simulink model "simulink6"  (R2025b)
settings: Solver=ode45  StartTime=0.0  StopTime=50  MaxStep=2^-5  RelTol=1e-3
settings Model: Creator=mizula  LastModifiedBy=mizula

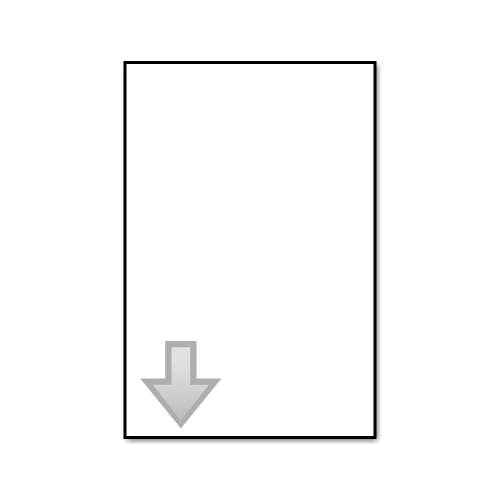
[thumbnail: Simulink's stored preview of the top-level diagram]
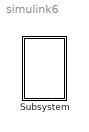
== system simulink6 ==
  Subsystem : Subsystem  mask{g=9.81, m1=1, m2=3, M=1, R=0.001, r0=2, th0=90, r1=0, th1=0}

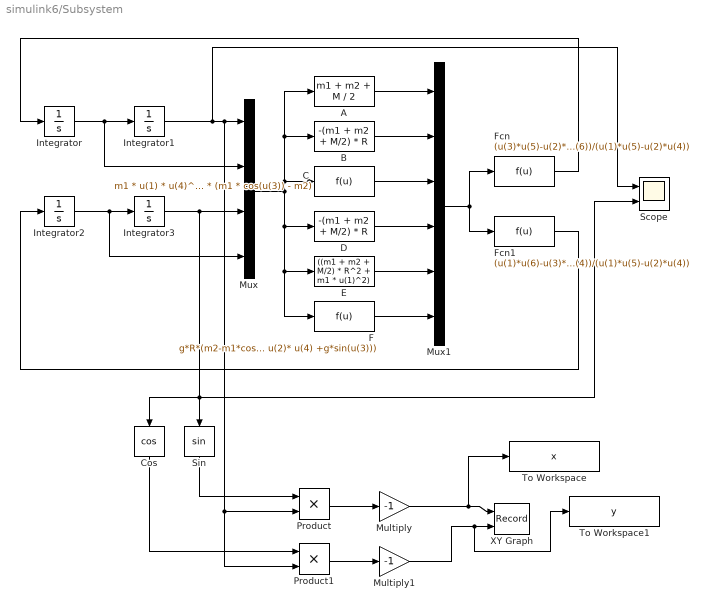
== system simulink6/Subsystem ==
  A : Fcn  Expr=m1 + m2 + M / 2
  B : Fcn  Expr=-(m1 + m2 + M/2) * R
  C : Fcn  Expr=m1 * u(1) * u(4)^2 + g * (m1 * cos(u(3)) - m2)
  Cos : Trigonometry  Operator=cos
  D : Fcn  Expr=-(m1 + m2 + M/2) * R
  E : Fcn  Expr=((m1 + m2 + M/2) * R^2 + m1 * u(1)^2)
  F : Fcn  Expr=g*R*(m2-m1*cos(u(3))) - m1*u(1)*(2 * u(2)* u(4) +g*sin(u(3)))
  Fcn : Fcn  Expr=(u(3)*u(5)-u(2)*u(6))/(u(1)*u(5)-u(2)*u(4))
  Fcn1 : Fcn  Expr=(u(1)*u(6)-u(3)*u(4))/(u(1)*u(5)-u(2)*u(4))
  Integrator : Integrator  InitialCondition=r1
  Integrator1 : Integrator  InitialCondition=r0
  Integrator2 : Integrator  InitialCondition=th1*pi/180
  Integrator3 : Integrator  InitialCondition=th0*pi/180
  Multiply : Gain  Gain=-1
  Multiply1 : Gain  Gain=-1
  Mux : Mux
  Mux1 : Mux  Inputs=6
  Product : Product
  Product1 : Product
  Scope : Scope  NumInputPorts=2
      settings: ActiveDisplayYMinimum=-1  ActiveDisplayYMaximum=1
  Sin : Trigonometry
  To Workspace : ToWorkspace  VariableName=x  SaveFormat=Timeseries  SampleTime=-1
  To Workspace1 : ToWorkspace  VariableName=y  SaveFormat=Timeseries  SampleTime=-1
  XY Graph : Record  NumPorts=2.0  FileSettingsInternal="{\"entries\":[{\"content\":{\"excelSettings\":{\"content\":{},\"type\":\"Streamout.ExcelSettings\"},\"parquetSettings\":{\"content\":{},\"type\":\"Streamout.ParquetSettings\"}},\"type\":\"Streamout.FileSettingStorage\",\"uuid\":\"\"}],\"packageUris\":[\"http:\\/\\/schema.mathworks.com\\/mf0\\/streamout_blocks\\/R2020a\"],\"version\":\"1.0\"}"  FrameSettings=[0, 0]  Layout=[1 1]  SignalsInternal="{\"entries\":[{\"content\":{\"signals\":[{\"content\":{\"blockPath\":[],\"dimensions\":[1],\"domain\":\"\",\"lineColor\":\"#a2142f\",\"plots\":[ 1 ],\"port\":1,\"sid\":[\"\"],\"signalID\":1,\"signalName\":\"Multiply\"},\"type\":\"RecordBlkView.Signal\",\"uuid\":\"\"},{\"content\":{\"blockPath\":[],\"dimensions\":[1],\"domain\":\"\",\"lineColor\":\"#139fff\",\"plots\":[ 1 ],\"port\":2,\"sid\":[\"\"],\"signalID\":2,\"signalName\":\"Multiply1\"},\"type\":\"RecordBlkView.Signal\",\"uuid\":\"\"}]},\"type\":\"RecordBlkView.InputSignals\",\"uuid\":\"\"}],\"packageUris\":[\"http:\\/\\/schema.mathworks.com\\/mf0\\/streamout_blocks\\/R2020a\"],\"version\":\"1.0\"}"  VisualizationBindings="{\"xyplotplugin\":{\"info\":[{\"series\":[{\"bindingParametersList\":[{\"parameter\":\"X-Axis\",\"signalID\":1,\"signalName\":\"Multiply\"},{\"parameter\":\"Y-Axis\",\"signalID\":2,\"signalName\":\"Multiply1\"}],\"seriesID\":0}],\"subplotID\":1}]}}"  CompatibilityTag=XY
  wires:
  Fcn1/1 -> Integrator2/1
  Sin/1 -> Product/1
  D/1 -> Mux1/4
  Multiply1/1 -> To Workspace1/1, XY Graph/2
  Multiply/1 -> To Workspace/1, XY Graph/1
  Integrator/1 -> Mux/2, Integrator1/1
  C/1 -> Mux1/3
  Integrator2/1 -> Mux/4, Integrator3/1
  A/1 -> Mux1/1
  Fcn/1 -> Integrator/1
  Product1/1 -> Multiply1/1
  Integrator1/1 -> Scope/1, Product1/2, Product/2, Mux/1
  Mux/1 -> A/1, B/1, C/1, E/1, F/1, D/1
  E/1 -> Mux1/5
  Integrator3/1 -> Scope/2, Sin/1, Cos/1, Mux/3
  F/1 -> Mux1/6
  B/1 -> Mux1/2
  Product/1 -> Multiply/1
  Cos/1 -> Product1/1
  Mux1/1 -> Fcn1/1, Fcn/1
